simulink model "power_igbtconv"  (Simulink 6.0)
settings: Solver=ode23tb  StartTime=0.0  StopTime=20e-3  RelTol=1e-3  AbsTol=1e-3
libraries: powerlib x7
settings Model: Creator=dkennedy  LastModifiedBy=batserve  ExtModeTrigMode=oneshot  ExtModeArmWhenConnect=off  ExtModeAutoUpdateStatusClock=off
settings DataIOCC: LimitDataPoints=off  SignalLoggingName=sigsOut
settings OptimizationCC: BlockReduction=off  BooleanDataType=off
settings DebuggingCC: SolverPrmCheckMsg=none
settings HardwareCC: TargetUnknown=on

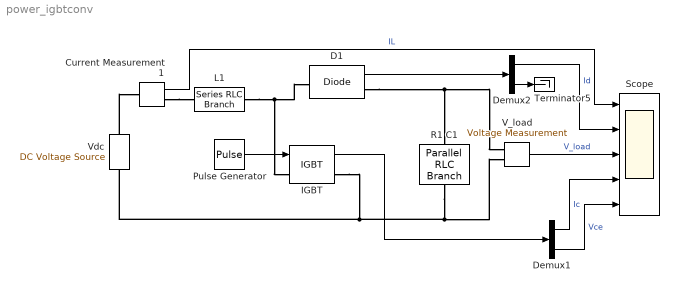
== system power_igbtconv ==
  Current Measurement1 : powerlib/Measurements/Current Measurement  Tag=PoWeRsYsTeMmEaSuReMeNt  PhasorSimulation=off  OutputType=Magnitude  PSBequivalent=0
  D1 : powerlib/Power Electronics/Diode  Ron=0.05  Lon=0.1e-6  Vf=0.8  IC=0  Rs=1e5  Cs=inf  Measurements=on
  Demux1 : Demux  Outputs=2
  Demux2 : Demux  Outputs=2
  IGBT : powerlib/Power Electronics/IGBT  Ron=0.01  Lon=1e-6  Vf=1  Tf=1e-6  Tt=1e-6  IC=0  Rs=10000  Cs=inf  Measurements=on
      settings: AttributesFormatString=\n
  L1 : powerlib/Elements/Series RLC Branch  PhysicalDomain=powersysdomain  SubClassName=unknown  LeftPortType=p1  RightPortType=p1  LConnTagsString=__new0  RConnTagsString=__new0  Resistance=0  Inductance=400e-6  Capacitance=inf  Measurements=None
  Pulse Generator : DiscretePulseGenerator  PulseType=Time based  Period=100e-6  PulseWidth=50
  R1 C1 : powerlib/Elements/Parallel RLC Branch  Orientation=down  PhysicalDomain=powersysdomain  SubClassName=unknown  LeftPortType=p1  RightPortType=p1  LConnTagsString=a  RConnTagsString=__new0  Resistance=50  Inductance=inf  Capacitance=25e-06  Measurements=None
  Scope : Scope  NumInputPorts=5
      settings: TimeRange=0.02  YMin=-10~0~0~0~0  YMax=70~70~400~70~700  SaveName=var  MaxDataPoints=50000
  Terminator5 : Terminator
  V_load : powerlib/Measurements/Voltage Measurement  Tag=PoWeRsYsTeMmEaSuReMeNt  PhasorSimulation=off  OutputType=Magnitude  PSBequivalent=0
  Vdc : powerlib/Electrical Sources/DC Voltage Source  Description=source block  Orientation=up  Amplitude=100  Measurements=None
      settings: AttributesFormatString=\n
  wires:
  Demux2/2 -> Terminator5/1
  Demux2/1 -> Scope/2  "Id"
  Demux1/1 -> Scope/4  "Ic"
  Demux1/2 -> Scope/5  "Vce"
  IGBT/1 -> Demux1/1
  Pulse Generator/1 -> IGBT/1
  Current Measurement1/1 -> Scope/1  "IL"
  D1/1 -> Demux2/1
  V_load/1 -> Scope/3  "V_load"
  connections:
  D1/RConn1 -- R1 C1/LConn1 -- V_load/LConn1
  R1 C1/RConn1 -- V_load/LConn2 -- Vdc/LConn1 -- IGBT/RConn1
  Current Measurement1/RConn1 -- L1/LConn1
  Vdc/RConn1 -- Current Measurement1/LConn1
  L1/RConn1 -- D1/LConn1 -- IGBT/LConn1
